simulink model "Orbit_Simulation"  (R2024a)
settings: Solver=FixedStepAuto  StartTime=t_start  StopTime=t_stop  FixedStep=t_step  RelTol=1e-3
values from neighbouring files (symbols this model uses):
  a = 1 / (2 / r_ECI - v_ECI^2 / Gm_Earth)    [ECI2OE.m]    (also in Orbit_Groundtrack.m = 7155.81)
  e = sqrt(1 - p / a)    [ECI2OE.m]    (also in Orbit_Groundtrack.m = 0.0001971)
  e_E = 0.0818    [Orbit_Groundtrack.m]
  incl = 86.403    [Orbit_Groundtrack.m]
  M_init = M_0    (= 267.074)    [Orbit_Groundtrack.m]
  MJD_init_UT1 = 60372    [Orbit_Groundtrack.m]
  n = sqrt(Gm_Earth / a^3)    [ECI2OE.m]    (also in Orbit_Groundtrack.m)
  Omega = Omega + 360    [ECI2OE.m]    (also in Orbit_Groundtrack.m = 230.875)
  omega = wrapTo360(u - nu)    [ECI2OE.m]    (also in Orbit_Groundtrack.m = 93.069)
  r_E = 6378.1    [Orbit_Groundtrack.m]
settings Model: Creator=jensr  LastModifiedBy=jensr
settings RTWCC: GPUComputeCapability=3.5

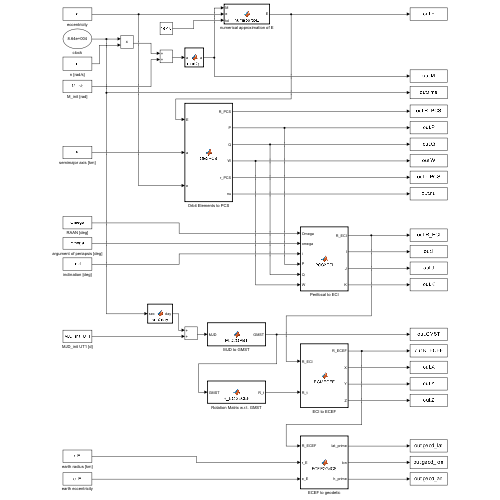
[thumbnail: Simulink's stored preview of the top-level diagram]
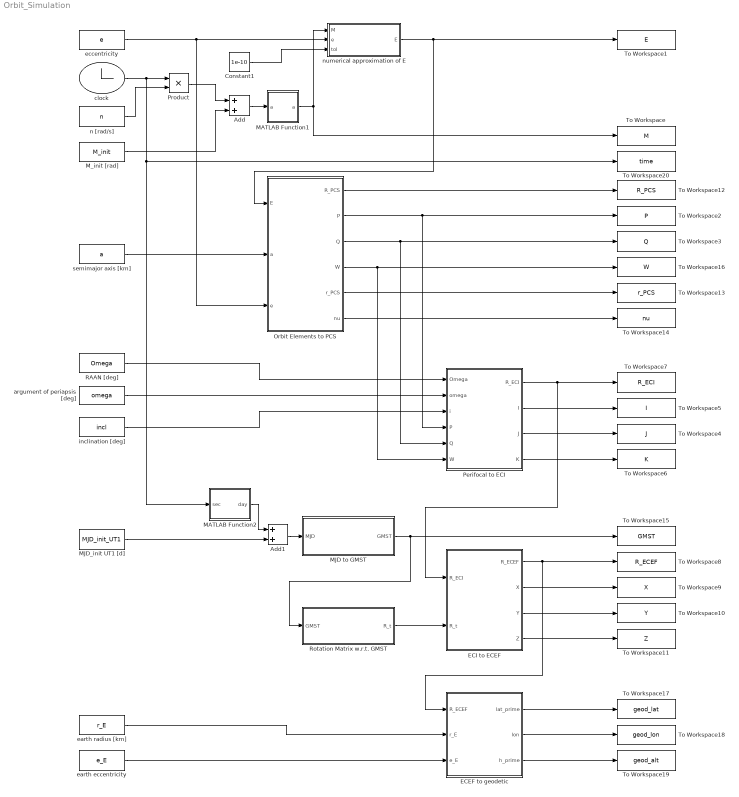
== system Orbit_Simulation ==
  Add : Sum
  Add1 : Sum
  Constant1 : Constant  Value=1e-10
  ECEF to geodetic : MATLAB Function  TreatAsAtomicUnit=on
  ECI to ECEF : MATLAB Function  TreatAsAtomicUnit=on
  MATLAB Function1 : MATLAB Function  TreatAsAtomicUnit=on
  MATLAB Function2 : MATLAB Function  TreatAsAtomicUnit=on
  MJD to GMST : MATLAB Function  TreatAsAtomicUnit=on
  MJD_init UT1 [d] : Constant  Value=MJD_init_UT1
  M_init [rad] : Constant  Value=M_init
  Orbit Elements to PCS : MATLAB Function  TreatAsAtomicUnit=on
  Perifocal to ECI : MATLAB Function  TreatAsAtomicUnit=on
  Product : Product
  RAAN [deg] : Constant  Value=Omega
  Rotation Matrix w.r.t. GMST : MATLAB Function  TreatAsAtomicUnit=on
  To Workspace : ToWorkspace  VariableName=M  SaveFormat=Timeseries  SampleTime=-1
  To Workspace1 : ToWorkspace  VariableName=E  SaveFormat=Timeseries  SampleTime=-1
  To Workspace10 : ToWorkspace  VariableName=Y  SaveFormat=Timeseries  SampleTime=-1
  To Workspace11 : ToWorkspace  VariableName=Z  SaveFormat=Timeseries  SampleTime=-1
  To Workspace12 : ToWorkspace  VariableName=R_PCS  SaveFormat=Timeseries  SampleTime=-1
  To Workspace13 : ToWorkspace  VariableName=r_PCS  SaveFormat=Timeseries  SampleTime=-1
  To Workspace14 : ToWorkspace  VariableName=nu  SaveFormat=Timeseries  SampleTime=-1
  To Workspace15 : ToWorkspace  VariableName=GMST  SaveFormat=Timeseries  SampleTime=-1
  To Workspace16 : ToWorkspace  VariableName=W  SaveFormat=Timeseries  SampleTime=-1
  To Workspace17 : ToWorkspace  VariableName=geod_lat  SaveFormat=Timeseries  SampleTime=-1
  To Workspace18 : ToWorkspace  VariableName=geod_lon  SaveFormat=Timeseries  SampleTime=-1
  To Workspace19 : ToWorkspace  VariableName=geod_alt  SaveFormat=Timeseries  SampleTime=-1
  To Workspace2 : ToWorkspace  VariableName=P  SaveFormat=Timeseries  SampleTime=-1
  To Workspace20 : ToWorkspace  VariableName=time  SaveFormat=Timeseries  SampleTime=-1
  To Workspace3 : ToWorkspace  VariableName=Q  SaveFormat=Timeseries  SampleTime=-1
  To Workspace4 : ToWorkspace  VariableName=J  SaveFormat=Timeseries  SampleTime=-1
  To Workspace5 : ToWorkspace  VariableName=I  SaveFormat=Timeseries  SampleTime=-1
  To Workspace6 : ToWorkspace  VariableName=K  SaveFormat=Timeseries  SampleTime=-1
  To Workspace7 : ToWorkspace  VariableName=R_ECI  SaveFormat=Timeseries  SampleTime=-1
  To Workspace8 : ToWorkspace  VariableName=R_ECEF  SaveFormat=Timeseries  SampleTime=-1
  To Workspace9 : ToWorkspace  VariableName=X  SaveFormat=Timeseries  SampleTime=-1
  argument of periapsis [deg] : Constant  Value=omega
  clock : Clock
  earth eccentricity : Constant  Value=e_E
  earth radius [km] : Constant  Value=r_E
  eccentricity : Constant  Value=e
  inclination [deg] : Constant  Value=incl
  n [rad/s] : Constant  Value=n
  numerical approximation of E : MATLAB Function  TreatAsAtomicUnit=on
  semimajor axis [km] : Constant  Value=a
  wires:
  n [rad/s]/1 -> Product/2
  M_init [rad]/1 -> Add/2
  Product/1 -> Add/1
  MATLAB Function1/1(a) -> numerical approximation of E/1(M), To Workspace/1
  Constant1/1 -> numerical approximation of E/3(tol)
  numerical approximation of E/1(E) -> To Workspace1/1, Orbit Elements to PCS/1(E)
  Orbit Elements to PCS/3(Q) -> Perifocal to ECI/5(Q), To Workspace3/1
  Orbit Elements to PCS/2(P) -> Perifocal to ECI/4(P), To Workspace2/1
  eccentricity/1 -> numerical approximation of E/2(e), Orbit Elements to PCS/3(e)
  Perifocal to ECI/3(J) -> To Workspace4/1
  Perifocal to ECI/2(I) -> To Workspace5/1
  Perifocal to ECI/4(K) -> To Workspace6/1
  RAAN [deg]/1 -> Perifocal to ECI/1(Omega)
  argument of periapsis [deg]/1 -> Perifocal to ECI/2(omega)
  inclination [deg]/1 -> Perifocal to ECI/3(i)
  Perifocal to ECI/1(R_ECI) -> ECI to ECEF/1(R_ECI), To Workspace7/1
  ECI to ECEF/1(R_ECEF) -> ECEF to geodetic/1(R_ECEF), To Workspace8/1
  ECI to ECEF/2(X) -> To Workspace9/1
  ECI to ECEF/3(Y) -> To Workspace10/1
  ECI to ECEF/4(Z) -> To Workspace11/1
  MJD_init UT1 [d]/1 -> Add1/2
  Rotation Matrix w.r.t. GMST/1(R_t) -> ECI to ECEF/2(R_t)
  semimajor axis [km]/1 -> Orbit Elements to PCS/2(a)
  Orbit Elements to PCS/1(R_PCS) -> To Workspace12/1
  Orbit Elements to PCS/4(W) -> Perifocal to ECI/6(W), To Workspace16/1
  Orbit Elements to PCS/5(r_PCS) -> To Workspace13/1
  Orbit Elements to PCS/6(nu) -> To Workspace14/1
  MJD to GMST/1(GMST) -> Rotation Matrix w.r.t. GMST/1(GMST), To Workspace15/1
  Add1/1 -> MJD to GMST/1(MJD)
  MATLAB Function2/1(day) -> Add1/1
  Add/1 -> MATLAB Function1/1("a ")
  earth radius [km]/1 -> ECEF to geodetic/2(r_E)
  ECEF to geodetic/1(lat_prime) -> To Workspace17/1
  ECEF to geodetic/2(lon) -> To Workspace18/1
  ECEF to geodetic/3(h_prime) -> To Workspace19/1
  earth eccentricity/1 -> ECEF to geodetic/3(e_E)
  clock/1 -> Product/1, To Workspace20/1, MATLAB Function2/1(sec)

== matlab function Orbit_Simulation/Perifocal to ECI ==
  data: R_ECI output; Omega input; omega input; i input; P input; I output; Q input; J output; K output; W input
function [R_ECI, I, J , K] = PCS2ECI(Omega, omega, i, P, Q, W)
    R_PCS = [P; Q; W];

    R_ECI = R_zd(-Omega) * R_xd(-i) * R_zd(-omega) * R_PCS;

    I = R_ECI(1);
    J = R_ECI(2);
    K = R_ECI(3);
end

function R_x = R_xd(a)
    R_x = [1, 0, 0; 0, cosd(a), sind(a); 0, -sind(a), cosd(a)];
end

function R_z = R_zd(a)
    R_z = [cosd(a), sind(a), 0; -sind(a), cosd(a), 0; 0, 0, 1];
end

== matlab function Orbit_Simulation/numerical approximation of E ==
  data: M input; E output; e input; tol input
function E  = numapproxE(M, e, tol)
    E = pi;
    i = 1;

    while 1
        delta = - (E - e * sin(E) - M) / (1 - e * cos(E));
        E = E + delta;

        i = i + 1;

        if abs(delta) <= tol || i > 20
            break
        end
    end
end

== matlab function Orbit_Simulation/ECI to ECEF ==
  data: R_ECI input; R_t input; R_ECEF output; X output; Y output; Z output
function [R_ECEF, X, Y, Z] = ECI2ECEF(R_ECI, R_t)
    R_ECEF = R_t * R_ECI;
    X = R_ECEF(1);
    Y = R_ECEF(2);
    Z = R_ECEF(3);
end

== matlab function Orbit_Simulation/Rotation Matrix w.r.t. GMST ==
  data: GMST input; R_t output
function R_t = R_ECI2ECEF(GMST)
    R_t = [cosd(GMST), sind(GMST), 0; -sind(GMST), cosd(GMST), 0; 0, 0, 1];
end

== matlab function Orbit_Simulation/Orbit Elements to PCS ==
  data: R_PCS output; E input; P output; a input; e input; Q output; W output; r_PCS output; nu output
function [R_PCS, P, Q, W, r_PCS, nu] = OE2PCS(E, a, e)
   P = a * (cos(E) - e);
   Q = a * sqrt(1 - e^2) * sin(E);
   W = 0;

   R_PCS = [P; Q; W];
   
   r_PCS = a * (1 - e * cos(E));
   nu = acosd(P / r_PCS);
end

== matlab function Orbit_Simulation/MJD to GMST ==
  data: GMST output; MJD input
function GMST  = MJD2GMST(MJD)
    d = MJD - 51544.5;
    GMST = 280.4606 + 360.9856473 * d;
    GMST = mod(GMST, 360);
end

== matlab function Orbit_Simulation/MATLAB Function1 ==
  data: a input; a output
function a  = mod2pi(a)
    a = mod(a, 2*pi);
end

== matlab function Orbit_Simulation/ECEF to geodetic ==
  data: R_ECEF input; r_E input; lat_prime output; e_E input; lon output; h_prime output
function [lat_prime, lon, h_prime] = ECEF2GdCS(R_ECEF, r_E, e_E)
% Converts a position vector in ECEF into geodetic coordinate system
    r_XY = sqrt(R_ECEF(1)^2 + R_ECEF(2)^2);

    % 1) longitude from geocentric longitude
    if R_ECEF(1) == 0 && R_ECEF(2) == 0
        lon = 0;
    else
        lon = atan2d(R_ECEF(2), R_ECEF(1));
    end
    
    % 2) geocentric latitude as first guess for geodetic latitude
    lat_prime = asind(R_ECEF(3) / sqrt(R_ECEF(1)^2 + R_ECEF(2)^2 + R_ECEF(3)^2));

    i = 1;
    while 1
        % 3) modified radius of curvature
        N = r_E / sqrt(1 - e_E^2 * sind(lat_prime)^2);

        % 4) update geodetic latitude
        lat_new = atan2d((R_ECEF(3) + N * e_E^2 * sind(lat_prime)), r_XY);
        delta = lat_prime - lat_new;
        lat_prime = lat_new;
                
        i = i + 1;
        
        % 5) check tolerance
        if abs(delta) <= 1e-10 || i > 20
            break
        end
    end

    % 6) compute altitude
    h_prime = r_XY / cosd(lat_prime) - N;
end

== matlab function Orbit_Simulation/MATLAB Function2 ==
  data: sec input; day output
function day = sec2day(sec)
    day = sec / 24 / 60 / 60;
end
